simulink model "Question4_system"  (R2020b)
settings: Solver=ode45  StartTime=0.0  StopTime=100  MaxStep=0.001  RelTol=1e-3
settings Model: Creator=sneha  LastModifiedBy=sneha

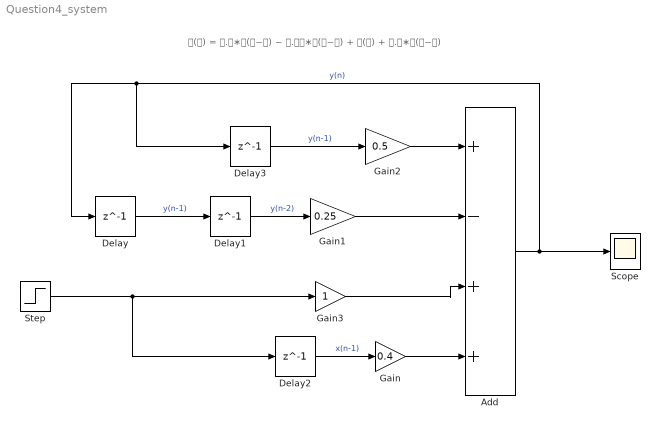
== system Question4_system ==
  note: 𝐲(𝐧) = 𝟎.𝟓∗𝐲(𝐧−𝟏) − 𝟎.𝟐𝟓∗𝐲(𝐧−𝟐) + 𝐱(𝐧) + 𝟎.𝟒∗𝐱(𝐧−𝟏)
  Add : Sum  Inputs=+-++
  Delay{,1..3} (4 alike) : Delay  DelayLength=1
  Gain : Gain  Gain=0.4
  Gain1 : Gain  Gain=0.25
  Gain2 : Gain  Gain=0.5
  Gain3 : Gain
  Scope : Scope
  Step : Step  SampleTime=0
  wires:
  Add/1 -> Delay3/1, Delay/1, Scope/1  "y(n)"
  Delay3/1 -> Gain2/1  "y(n-1)"
  Gain/1 -> Add/4
  Delay/1 -> Delay1/1  "y(n-1)"
  Gain1/1 -> Add/2
  Delay2/1 -> Gain/1  "x(n-1)"
  Delay1/1 -> Gain1/1  "y(n-2)"
  Gain2/1 -> Add/1
  Step/1 -> Delay2/1, Gain3/1
  Gain3/1 -> Add/3
